simulink model "dpt"  (R2023a)
settings: Solver=VariableStepAuto  StartTime=0.0  StopTime=7  RelTol=1e-3
values from neighbouring files (symbols this model uses):
  Cm = 1.3    [const.m]
  Cw = 3.15    [const.m]
  f = 0.001    [const.m]
  J = 7e-6    (= 7e-06)    [const.m]
  La = 0.0015    [const.m]
  Lew = 0.013    [const.m]
  R = 8    [const.m]
settings Model: Creator=mrrom  LastModifiedBy=mrrom

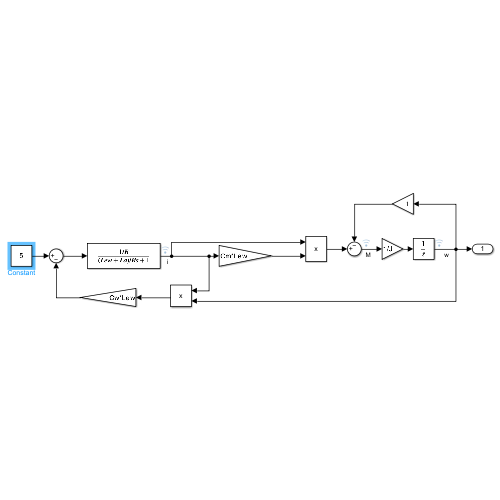
[thumbnail: Simulink's stored preview of the top-level diagram]
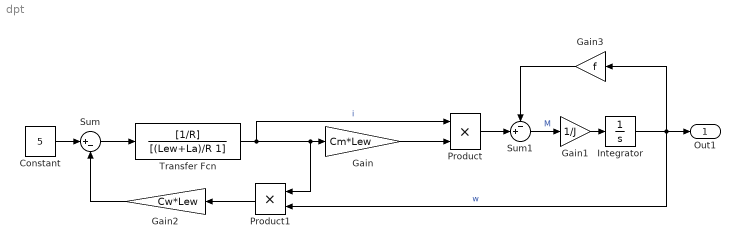
== system dpt ==
  Constant : Constant  Value=5
  Gain : Gain  Gain=Cm*Lew
  Gain1 : Gain  Gain=1/J
  Gain2 : Gain  Gain=Cw*Lew
  Gain3 : Gain  Gain=f
  Integrator : Integrator
  Product : Product
  Product1 : Product
  Sum : Sum  Inputs=|+-
  Sum1 : Sum  Inputs=-+|
  Transfer Fcn : TransferFcn  Numerator=[1/R]  Denominator=[(Lew+La)/R 1]
  Out1 : Outport
  wires:
  Sum/1 -> Transfer Fcn/1
  Constant/1 -> Sum/1
  Transfer Fcn/1 -> Product1/1, Gain/1, Product/1  "i"
  Gain/1 -> Product/2
  Gain2/1 -> Sum/2
  Product1/1 -> Gain2/1
  Gain1/1 -> Integrator/1
  Integrator/1 -> Product1/2, Out1/1, Gain3/1  "w"
  Product/1 -> Sum1/2
  Sum1/1 -> Gain1/1  "M"
  Gain3/1 -> Sum1/1
